simulink model "w2_prob2_214869"  (R2020a)
settings: Solver=ode23  StartTime=0.0  StopTime=10.0  RelTol=1e-3
values from neighbouring files (symbols this model uses):
  be = 2.0    [prob2.sldd]
  bv = 1.0    [prob2.sldd]
  le = 1.0    [prob2.sldd]
  lv = 5.0    [prob2.sldd]
settings Model: DataDictionary=prob2.sldd  Creator=sonal  LastModifiedBy=sonal

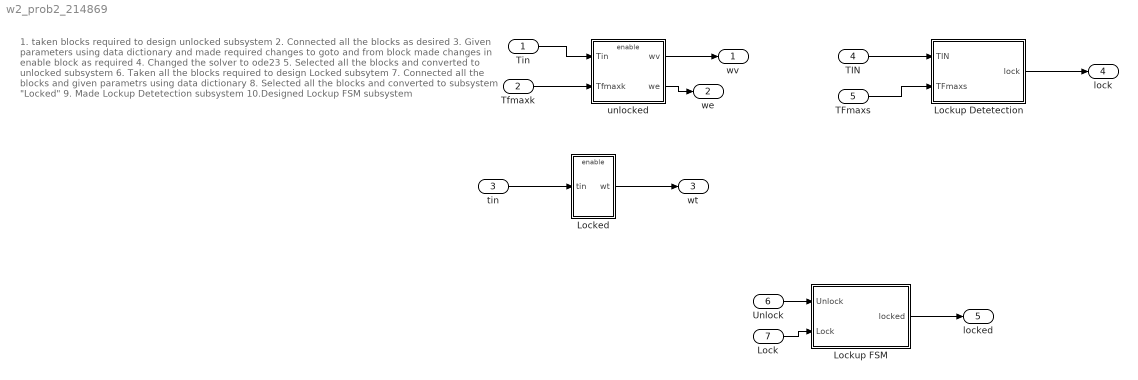
== system w2_prob2_214869 ==
  note: 1. taken blocks required to design unlocked subsystem
      | 2. Connected all the blocks as desired
      | 3. Given parameters using data dictionary
      | and made required changes to goto and from block
      | made changes in enable block as required
      | 4. Changed the solver to ode23
      | 5. Selected all the blocks and converted to unlocked subsystem
      | 6. Taken all the blocks required to design Locked subsytem
      | 7. Connected all the blocks and given parametrs using data dictionary
      | 8. Selected all the blocks and converted to subsystem "Locked"
      | 9. Made Lockup Detetection subsystem
      | 10.Designed Lockup FSM subsystem
  Tin : Inport
  Tfmaxk : Inport  Port=2
  tin : Inport  Port=3
  TIN : Inport  Port=4
  TFmaxs : Inport  Port=5
  Unlock : Inport  Port=6
  Lock : Inport  Port=7
  Locked : Subsystem
  Lockup Detetection : Subsystem
  Lockup FSM : Subsystem
  unlocked : Subsystem
  wv : Outport
  we : Outport  Port=2
  wt : Outport  Port=3
  lock : Outport  Port=4
  locked : Outport  Port=5
  wires:
  Tin/1 -> unlocked/1(Tin)
  Tfmaxk/1 -> unlocked/2(Tfmaxk)
  unlocked/1(wv) -> wv/1
  unlocked/2(we) -> we/1
  tin/1 -> Locked/1(tin)
  Locked/1(wt) -> wt/1
  TIN/1 -> Lockup Detetection/1(TIN)
  TFmaxs/1 -> Lockup Detetection/2(TFmaxs)
  Lockup Detetection/1(lock) -> lock/1
  Unlock/1 -> Lockup FSM/1(Unlock)
  Lock/1 -> Lockup FSM/2(Lock)
  Lockup FSM/1(locked) -> locked/1

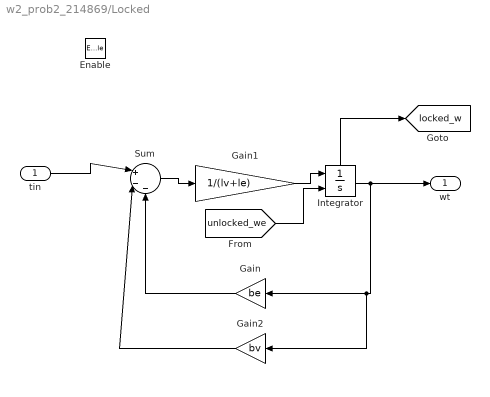
== system w2_prob2_214869/Locked ==
  tin : Inport
  Enable : EnablePort  StatesWhenEnabling=reset
  Gain : Gain  Gain=be
  Gain1 : Gain  Gain=1/(lv+le)
  Gain2 : Gain  Gain=bv
  Integrator : Integrator  InitialConditionSource=external  ShowStatePort=on
  Sum : Sum  Inputs=|+--
  wt : Outport
  tag scope: locked_w=global
  wires:
  Sum/1 -> Gain1/1
  Integrator/1 -> wt/1, Gain2/1, Gain/1
  Gain/1 -> Sum/3
  Integrator/State -> [locked_w]
  Gain2/1 -> Sum/2
  [unlocked_we] -> Integrator/2
  Gain1/1 -> Integrator/1
  tin/1 -> Sum/1

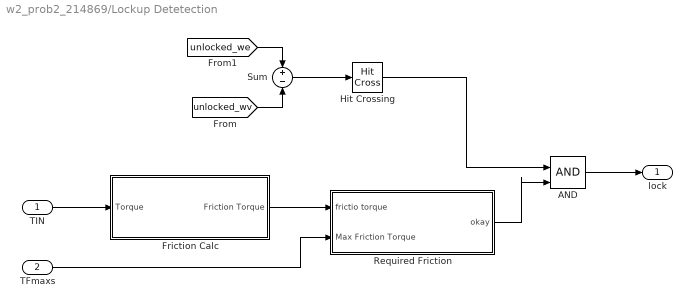
== system w2_prob2_214869/Lockup Detetection ==
  TIN : Inport
  TFmaxs : Inport  Port=2
  AND : Logic  IconShape=distinctive  AllPortsSameDT=off  OutDataTypeStr=boolean
  Friction Calc : Subsystem
  Hit Crossing : HitCross
  Required Friction : Subsystem
  Sum : Sum  Inputs=+-
  lock : Outport
  wires:
  Hit Crossing/1 -> AND/1
  Required Friction/1(okay) -> AND/2
  [unlocked_we] -> Sum/1
  Sum/1 -> Hit Crossing/1
  [unlocked_wv] -> Sum/2
  AND/1 -> lock/1
  Friction Calc/1(Friction Torque) -> Required Friction/1(frictio torque)
  TFmaxs/1 -> Required Friction/2(Max Friction Torque)
  TIN/1 -> Friction Calc/1(Torque)

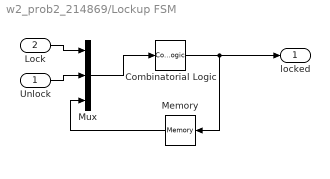
== system w2_prob2_214869/Lockup FSM ==
  Unlock : Inport
  Lock : Inport  Port=2
  Combinatorial Logic : CombinatorialLogic  TruthTable=[0;1;0;0;1;1;1;0]
  Memory : Memory
  Mux : Mux  Inputs=3
  locked : Outport
  wires:
  Combinatorial Logic/1 -> locked/1, Memory/1
  Unlock/1 -> Mux/2
  Mux/1 -> Combinatorial Logic/1
  Lock/1 -> Mux/1
  Memory/1 -> Mux/3

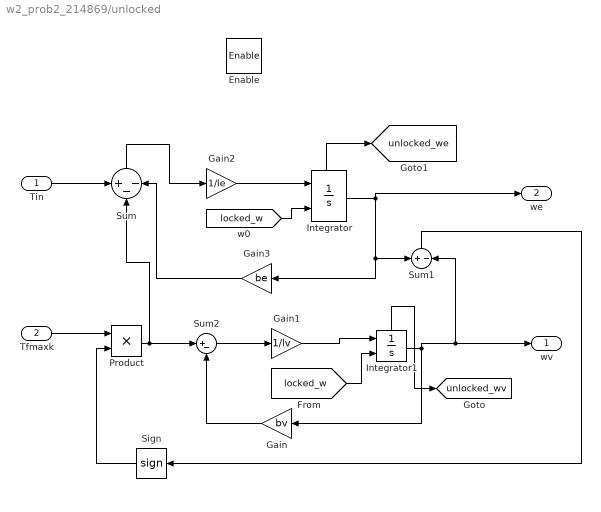
== system w2_prob2_214869/unlocked ==
  Tin : Inport
  Tfmaxk : Inport  Port=2
  Enable : EnablePort  StatesWhenEnabling=reset
  Gain : Gain  Gain=bv
  Gain1 : Gain  Gain=1/lv
  Gain2 : Gain  Gain=1/le
  Gain3 : Gain  Gain=be
  Integrator : Integrator  InitialConditionSource=external  ShowStatePort=on
  Integrator1 : Integrator  InitialConditionSource=external  ShowStatePort=on
  Product : Product
  Sign : Signum
  Sum : Sum  Inputs=+--
  Sum1 : Sum  Inputs=+-
  Sum2 : Sum  Inputs=|+-
  wv : Outport
  we : Outport  Port=2
  tag scope: unlocked_we=global, unlocked_wv=global
  wires:
  Gain2/1 -> Integrator/1
  Gain/1 -> Sum2/2
  Integrator1/State -> [unlocked_wv]
  Product/1 -> Sum2/1, Sum/2
  Sum1/1 -> Sign/1
  Integrator1/1 -> wv/1, Sum1/2, Gain/1
  [locked_w] -> Integrator/2
  [locked_w] -> Integrator1/2
  Integrator/1 -> we/1, Sum1/1, Gain3/1
  Gain3/1 -> Sum/3
  Tfmaxk/1 -> Product/1
  Sign/1 -> Product/2
  Sum2/1 -> Gain1/1
  Tin/1 -> Sum/1
  Integrator/State -> [unlocked_we]
  Sum/1 -> Gain2/1
  Gain1/1 -> Integrator1/1

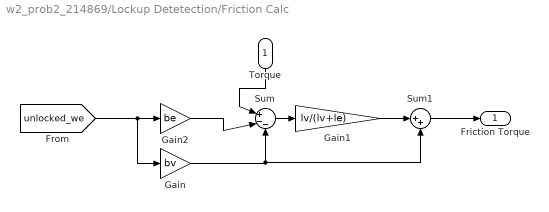
== system w2_prob2_214869/Lockup Detetection/Friction Calc ==
  Torque : Inport
  Gain : Gain  Gain=bv
  Gain1 : Gain  Gain=lv/(lv+le)
  Gain2 : Gain  Gain=be
  Sum : Sum  Inputs=|+--
  Sum1 : Sum  Inputs=|++
  Friction Torque : Outport
  wires:
  Sum/1 -> Gain1/1
  [unlocked_we] -> Gain/1, Gain2/1
  Gain1/1 -> Sum1/1
  Torque/1 -> Sum/1
  Sum1/1 -> Friction Torque/1
  Gain2/1 -> Sum/2
  Gain/1 -> Sum1/2, Sum/3

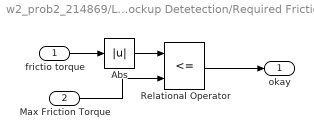
== system w2_prob2_214869/Lockup Detetection/Required Friction ==
  frictio torque : Inport
  Max Friction Torque : Inport  Port=2
  Abs : Abs
  Relational Operator : RelationalOperator  Operator=<=  OutDataTypeStr=boolean  RndMeth=Simplest
  okay : Outport
  wires:
  Max Friction Torque/1 -> Relational Operator/2
  Relational Operator/1 -> okay/1
  Abs/1 -> Relational Operator/1
  frictio torque/1 -> Abs/1
